simulink library "mysharedTrackingLibrary"  (R2023b)
settings: Solver=VariableStepAuto  StartTime=0.0  StopTime=10.0  RelTol=1e-3
undefined symbols (not defined in the file or in its folder): p
libraries: $bdroot x3
(part 2 of 2)

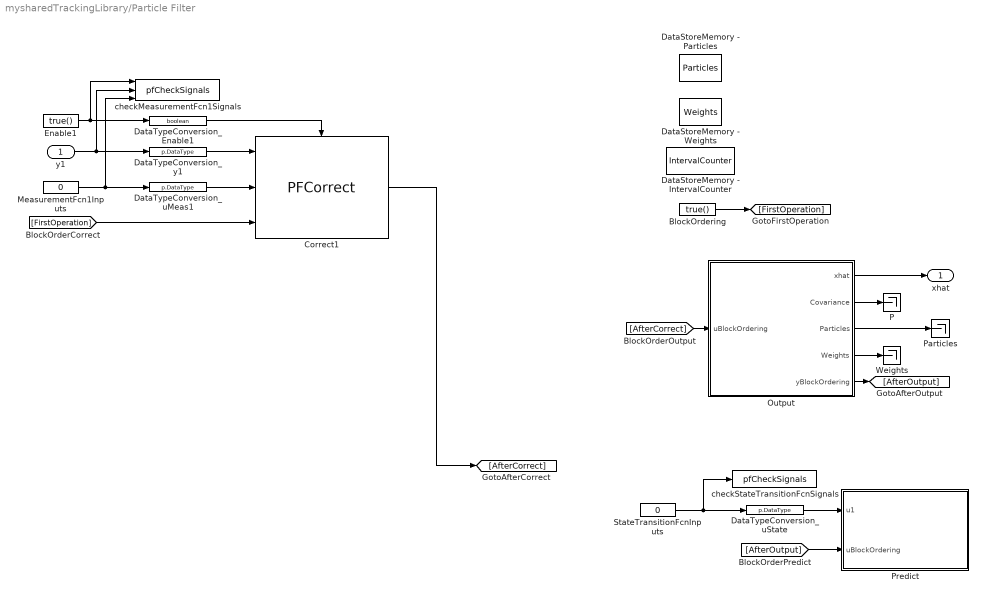
== system mysharedTrackingLibrary/Particle Filter ==
  y1 : Inport
  BlockOrdering : Constant  Value=true()  OutDataTypeStr=boolean
  Correct1 : $bdroot/Extras/PFCorrect  ProcessedMaskData=p
  DataStoreMemory - IntervalCounter : DataStoreMemory  DataStoreName=IntervalCounter  VectorParams1D=off  ShowAdditionalParam=off  OutDataTypeStr=p.DataType
  DataStoreMemory - Particles : DataStoreMemory  DataStoreName=Particles  InitialValue=p.Particles  VectorParams1D=off  ShowAdditionalParam=off  OutDataTypeStr=p.DataType
  DataStoreMemory - Weights : DataStoreMemory  DataStoreName=Weights  InitialValue=p.Weights  VectorParams1D=off  ShowAdditionalParam=off  OutDataTypeStr=p.DataType
  DataTypeConversion_Enable1 : DataTypeConversion  OutDataTypeStr=boolean  SaturateOnIntegerOverflow=off  RndMeth=Floor
  DataTypeConversion_uMeas1 : DataTypeConversion  OutDataTypeStr=p.DataType  SaturateOnIntegerOverflow=off  RndMeth=Floor
  DataTypeConversion_uState : DataTypeConversion  OutDataTypeStr=p.DataType  SaturateOnIntegerOverflow=off  RndMeth=Floor
  DataTypeConversion_y1 : DataTypeConversion  OutDataTypeStr=p.DataType  SaturateOnIntegerOverflow=off  RndMeth=Floor
  Enable1 : Constant  Value=true()  SampleTime=p.SampleTimes.MeasurementFcn(1)
  MeasurementFcn1Inputs : Constant  Value=0  OutDataTypeStr=p.DataType  SampleTime=p.SampleTimes.MeasurementFcn(1)
  Output : Subsystem  TreatAsAtomicUnit=on  SystemSampleTime=p.SampleTimes.Output  mask{ProcessedMaskData=p}
      mask init:
      | if strcmp(get_param(bdroot,'SimulationStatus'),'stopped')
      |     pOutputs = [];
      | else
      |     pOutputs = ...
      |         matlabshared.tracking.internal.blocks.maskInitializationFcnPFOutputs(ProcessedMaskData);
      | end
  P : Terminator
  Particles : Terminator
  Predict : Subsystem  TreatAsAtomicUnit=on  SystemSampleTime=p.SampleTimes.StateTransitionFcn  mask(PFPredict){ProcessedMaskData=p}
      mask init:
      | if strcmp(get_param(bdroot,'SimulationStatus'),'stopped')
      |     pS = [];
      |     SampleTime = [];
      |     DataType = [];
      |     SLFcnsToRegister = {};
      | else
      |     [pS,SampleTime] = ...
      |         matlabshared.tracking.internal.blocks.maskInitializationFcnPFPredictor(ProcessedMaskData);
      |     [DataType,SLFcnsToRegister] = ...
      |         matlabshared.tracking.internal.blocks.maskInitializationFcnRegisterSLFcn(ProcessedMaskData, pS);
      | end
  StateTransitionFcnInputs : Constant  Value=0  OutDataTypeStr=p.DataType  SampleTime=p.SampleTimes.StateTransitionFcn
  Weights : Terminator
  checkMeasurementFcn1Signals : S-Function  FunctionName=pfCheckSignals  Parameters=signalCheck.BlockPath, signalCheck.MeasurementFcn{1}.PortNames, signalCheck.MeasurementFcn{1}.SampleTime, signalCheck.DataType, signalCheck.MeasurementFcn{1}.PortDimensions  SFunctionDeploymentMode=off  EnableBusSupport=off
  checkStateTransitionFcnSignals : S-Function  FunctionName=pfCheckSignals  Parameters=signalCheck.BlockPath, signalCheck.StateTransitionFcn.PortNames, signalCheck.StateTransitionFcn.SampleTime, signalCheck.DataType, signalCheck.StateTransitionFcn.PortDimensions  SFunctionDeploymentMode=off  EnableBusSupport=off
  xhat : Outport  VectorParamsAs1DForOutWhenUnconnected=off
  wires:
  [AfterCorrect] -> Output/1(uBlockOrdering)
  Correct1/1 -> [AfterCorrect]
  [AfterOutput] -> Predict/2(uBlockOrdering)
  BlockOrdering/1 -> [FirstOperation]
  [FirstOperation] -> Correct1/3
  DataTypeConversion_y1/1 -> Correct1/1
  DataTypeConversion_uMeas1/1 -> Correct1/2
  Enable1/1 -> checkMeasurementFcn1Signals/1, DataTypeConversion_Enable1/1
  StateTransitionFcnInputs/1 -> checkStateTransitionFcnSignals/1, DataTypeConversion_uState/1
  MeasurementFcn1Inputs/1 -> checkMeasurementFcn1Signals/3, DataTypeConversion_uMeas1/1
  DataTypeConversion_uState/1 -> Predict/1(u1)
  DataTypeConversion_Enable1/1 -> Correct1/Enable
  Output/5(yBlockOrdering) -> [AfterOutput]
  Output/1(xhat) -> xhat/1
  Output/3(Particles) -> Particles/1
  Output/4(Weights) -> Weights/1
  Output/2(Covariance) -> P/1
  y1/1 -> DataTypeConversion_y1/1, checkMeasurementFcn1Signals/2

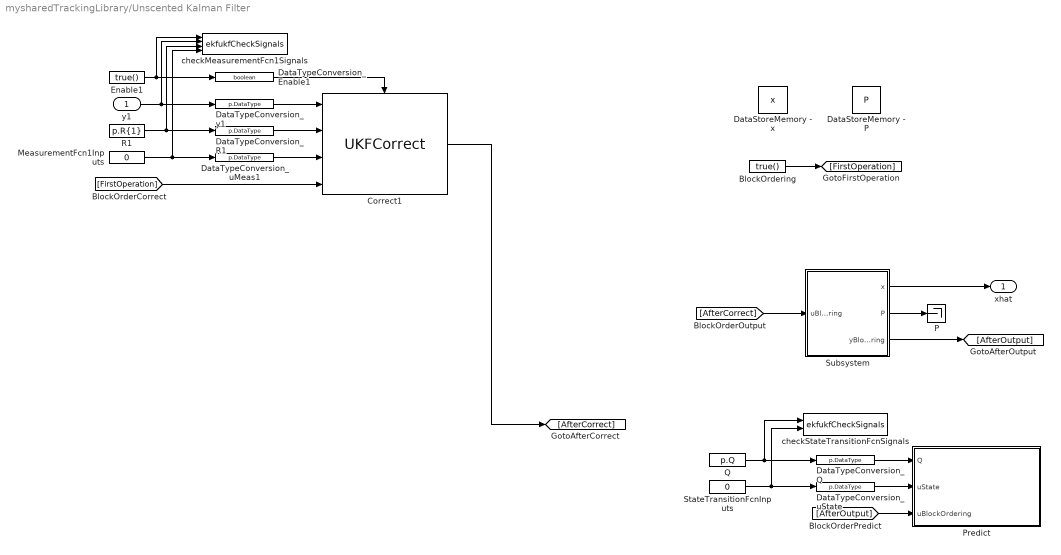
== system mysharedTrackingLibrary/Unscented Kalman Filter ==
  y1 : Inport
  BlockOrdering : Constant  Value=true()  OutDataTypeStr=boolean
  Correct1 : $bdroot/Extras/UKFCorrect  ProcessedMaskData=p
  DataStoreMemory - P : DataStoreMemory  DataStoreName=P  InitialValue=p.InitialCovariance  ShowAdditionalParam=off  OutDataTypeStr=p.DataType
  DataStoreMemory - x : DataStoreMemory  DataStoreName=x  InitialValue=p.InitialState  ShowAdditionalParam=off  OutDataTypeStr=p.DataType
  DataTypeConversion_Enable1 : DataTypeConversion  OutDataTypeStr=boolean  SaturateOnIntegerOverflow=off  RndMeth=Floor
  DataTypeConversion_Q : DataTypeConversion  OutDataTypeStr=p.DataType  SaturateOnIntegerOverflow=off  RndMeth=Floor
  DataTypeConversion_R1 : DataTypeConversion  OutDataTypeStr=p.DataType  SaturateOnIntegerOverflow=off  RndMeth=Floor
  DataTypeConversion_uMeas1 : DataTypeConversion  OutDataTypeStr=p.DataType  SaturateOnIntegerOverflow=off  RndMeth=Floor
  DataTypeConversion_uState : DataTypeConversion  OutDataTypeStr=p.DataType  SaturateOnIntegerOverflow=off  RndMeth=Floor
  DataTypeConversion_y1 : DataTypeConversion  OutDataTypeStr=p.DataType  SaturateOnIntegerOverflow=off  RndMeth=Floor
  Enable1 : Constant  Value=true()  SampleTime=p.SampleTimes.MeasurementFcn(1)
  MeasurementFcn1Inputs : Constant  Value=0  OutDataTypeStr=p.DataType  SampleTime=p.SampleTimes.MeasurementFcn(1)
  P : Terminator
  Predict : Subsystem  TreatAsAtomicUnit=on  SystemSampleTime=p.SampleTimes.StateTransitionFcn  mask(UKFPredict){ProcessedMaskData=p}
      mask init:
      | if strcmp(get_param(bdroot,'SimulationStatus'),'stopped')
      |     pS = [];
      |     SampleTime = [];
      |     DataType = [];
      |     SLFcnsToRegister = {};
      | else
      |     [pS,SampleTime] = ...
      |         matlabshared.tracking.internal.blocks.maskInitializationFcnUKFPredictor(ProcessedMaskData);
      |     [DataType,SLFcnsToRegister] = ...
      |         matlabshared.tracking.internal.blocks.maskInitializationFcnRegisterSLFcn(ProcessedMaskData, pS);
      | end
  Q : Constant  Value=p.Q  SampleTime=p.SampleTimes.StateTransitionFcn
  R1 : Constant  Value=p.R{1}  SampleTime=p.SampleTimes.MeasurementFcn(1)
  StateTransitionFcnInputs : Constant  Value=0  OutDataTypeStr=p.DataType  SampleTime=p.SampleTimes.StateTransitionFcn
  Subsystem : Subsystem  TreatAsAtomicUnit=on  SystemSampleTime=p.SampleTimes.Output
  checkMeasurementFcn1Signals : S-Function  FunctionName=ekfukfCheckSignals  Parameters=signalCheck.BlockPath, signalCheck.MeasurementFcn{1}.PortNames, signalCheck.MeasurementFcn{1}.SampleTime, signalCheck.DataType, signalCheck.MeasurementFcn{1}.PortDimensions, 1, signalCheck.MeasurementFcn{1}.HasAdditiveNoise  SFunctionDeploymentMode=off  EnableBusSupport=off
  checkStateTransitionFcnSignals : S-Function  FunctionName=ekfukfCheckSignals  Parameters=signalCheck.BlockPath, signalCheck.StateTransitionFcn.PortNames, signalCheck.StateTransitionFcn.SampleTime, signalCheck.DataType, signalCheck.StateTransitionFcn.PortDimensions, 0, signalCheck.StateTransitionFcn.HasAdditiveNoise  SFunctionDeploymentMode=off  EnableBusSupport=off
  xhat : Outport  VectorParamsAs1DForOutWhenUnconnected=off
  wires:
  [AfterOutput] -> Predict/3(uBlockOrdering)
  BlockOrdering/1 -> [FirstOperation]
  [FirstOperation] -> Correct1/4
  DataTypeConversion_y1/1 -> Correct1/1
  y1/1 -> checkMeasurementFcn1Signals/2, DataTypeConversion_y1/1
  R1/1 -> checkMeasurementFcn1Signals/3, DataTypeConversion_R1/1
  DataTypeConversion_uMeas1/1 -> Correct1/3
  Enable1/1 -> checkMeasurementFcn1Signals/1, DataTypeConversion_Enable1/1
  StateTransitionFcnInputs/1 -> checkStateTransitionFcnSignals/2, DataTypeConversion_uState/1
  MeasurementFcn1Inputs/1 -> checkMeasurementFcn1Signals/4, DataTypeConversion_uMeas1/1
  DataTypeConversion_R1/1 -> Correct1/2
  DataTypeConversion_uState/1 -> Predict/2(uState)
  Q/1 -> checkStateTransitionFcnSignals/1, DataTypeConversion_Q/1
  DataTypeConversion_Enable1/1 -> Correct1/Enable
  DataTypeConversion_Q/1 -> Predict/1(Q)
  [AfterCorrect] -> Subsystem/1(uBlockOrdering)
  Subsystem/1(x) -> xhat/1
  Subsystem/2(P) -> P/1
  Subsystem/3(yBlockOrdering) -> [AfterOutput]
  Correct1/1 -> [AfterCorrect]

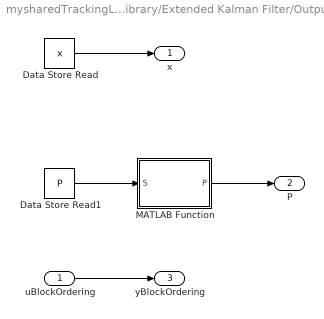
== system mysharedTrackingLibrary/Extended Kalman Filter/Output ==
  uBlockOrdering : Inport
  Data Store Read : DataStoreRead  DataStoreName=x  IndexOptions=Index vector (dialog)  Indices=1  OutputSizes=1
  Data Store Read1 : DataStoreRead  DataStoreName=P  IndexOptions=Index vector (dialog)  Indices=1  OutputSizes=1
  MATLAB Function : MATLAB Function  TreatAsAtomicUnit=on
  x : Outport  VectorParamsAs1DForOutWhenUnconnected=off
  P : Outport  Port=2  VectorParamsAs1DForOutWhenUnconnected=off
  yBlockOrdering : Outport  Port=3  VectorParamsAs1DForOutWhenUnconnected=off
  wires:
  Data Store Read/1 -> x/1
  Data Store Read1/1 -> MATLAB Function/1(S)
  uBlockOrdering/1 -> yBlockOrdering/1
  MATLAB Function/1(P) -> P/1

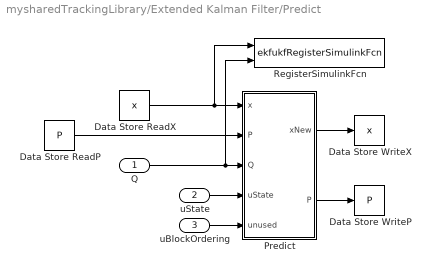
== system mysharedTrackingLibrary/Extended Kalman Filter/Predict ==
  Q : Inport  SampleTime=SampleTime
  uState : Inport  Port=2  SampleTime=SampleTime
  uBlockOrdering : Inport  Port=3  SampleTime=SampleTime
  Data Store WriteP : DataStoreWrite  DataStoreName=P  IndexOptions=Index vector (dialog)  Indices=1  OutputSizes=1
  Data Store WriteX : DataStoreWrite  DataStoreName=x  IndexOptions=Index vector (dialog)  Indices=1  OutputSizes=1
  Data Store ReadP : DataStoreRead  DataStoreName=P  IndexOptions=Index vector (dialog)  Indices=1  OutputSizes=1
  Data Store ReadX : DataStoreRead  DataStoreName=x  IndexOptions=Index vector (dialog)  Indices=1  OutputSizes=1
  Predict : MATLAB Function  TreatAsAtomicUnit=on
  RegisterSimulinkFcn : S-Function  FunctionName=ekfukfRegisterSimulinkFcn  Parameters=int32(2), 0, pS.HasAdditiveNoise, SampleTime, DataType, SLFcnsToRegister  SFunctionDeploymentMode=off  EnableBusSupport=off
  wires:
  Data Store ReadP/1 -> Predict/2("P ")
  Predict/2(P) -> Data Store WriteP/1
  Q/1 -> Predict/3(Q), RegisterSimulinkFcn/2
  Predict/1(xNew) -> Data Store WriteX/1
  Data Store ReadX/1 -> Predict/1(x), RegisterSimulinkFcn/1
  uBlockOrdering/1 -> Predict/5(unused)
  uState/1 -> Predict/4(uState)

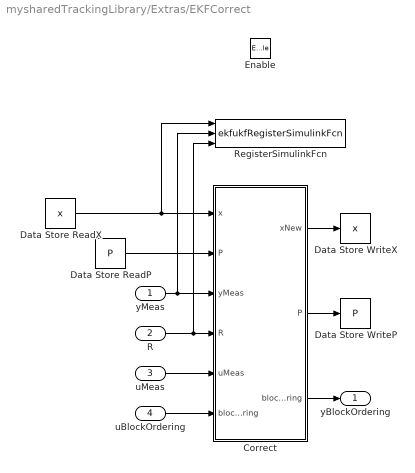
== system mysharedTrackingLibrary/Extras/EKFCorrect ==
  yMeas : Inport  SampleTime=SampleTime
  R : Inport  Port=2  SampleTime=SampleTime
  uMeas : Inport  Port=3  SampleTime=SampleTime
  uBlockOrdering : Inport  Port=4  SampleTime=SampleTime
  Enable : EnablePort
  Correct : MATLAB Function  TreatAsAtomicUnit=on
  Data Store ReadP : DataStoreRead  DataStoreName=P  IndexOptions=Index vector (dialog)  Indices=1  OutputSizes=1
  Data Store ReadX : DataStoreRead  DataStoreName=x  IndexOptions=Index vector (dialog)  Indices=1  OutputSizes=1
  Data Store WriteP : DataStoreWrite  DataStoreName=P  IndexOptions=Index vector (dialog)  Indices=1  OutputSizes=1
  Data Store WriteX : DataStoreWrite  DataStoreName=x  IndexOptions=Index vector (dialog)  Indices=1  OutputSizes=1
  RegisterSimulinkFcn : S-Function  FunctionName=ekfukfRegisterSimulinkFcn  Parameters=int32(3), 1, pM.HasAdditiveNoise, SampleTime, DataType, SLFcnsToRegister  SFunctionDeploymentMode=off  EnableBusSupport=off
  yBlockOrdering : Outport  VectorParamsAs1DForOutWhenUnconnected=off
  wires:
  Data Store ReadX/1 -> RegisterSimulinkFcn/1, Correct/1(x)
  Data Store ReadP/1 -> Correct/2("P ")
  Correct/2(P) -> Data Store WriteP/1
  yMeas/1 -> Correct/3(yMeas), RegisterSimulinkFcn/2
  R/1 -> Correct/4(R), RegisterSimulinkFcn/3
  Correct/1(xNew) -> Data Store WriteX/1
  Correct/3(blockOrdering) -> yBlockOrdering/1
  uBlockOrdering/1 -> Correct/6("blockOrdering ")
  uMeas/1 -> Correct/5(uMeas)

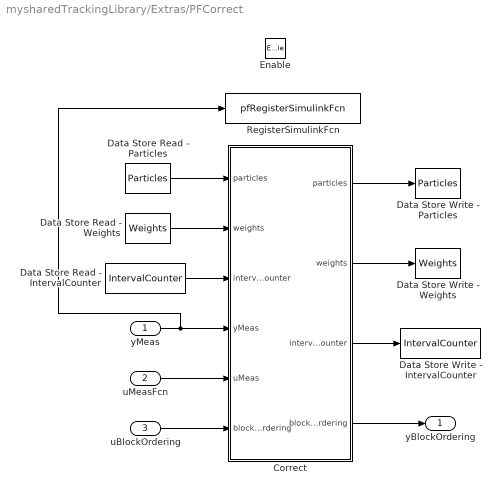
== system mysharedTrackingLibrary/Extras/PFCorrect ==
  yMeas : Inport  SampleTime=SampleTime
  uMeasFcn : Inport  Port=2  SampleTime=SampleTime
  uBlockOrdering : Inport  Port=3  SampleTime=SampleTime
  Enable : EnablePort
  Correct : MATLAB Function  TreatAsAtomicUnit=on
  Data Store Read - IntervalCounter : DataStoreRead  DataStoreName=IntervalCounter  IndexOptions=Index vector (dialog)  Indices=1  OutputSizes=1
  Data Store Read - Particles : DataStoreRead  DataStoreName=Particles  IndexOptions=Index vector (dialog)  Indices=1  OutputSizes=1
  Data Store Read - Weights : DataStoreRead  DataStoreName=Weights  IndexOptions=Index vector (dialog)  Indices=1  OutputSizes=1
  Data Store Write - IntervalCounter : DataStoreWrite  DataStoreName=IntervalCounter  IndexOptions=Index vector (dialog)  Indices=1  OutputSizes=1
  Data Store Write - Particles : DataStoreWrite  DataStoreName=Particles  IndexOptions=Index vector (dialog)  Indices=1  OutputSizes=1
  Data Store Write - Weights : DataStoreWrite  DataStoreName=Weights  IndexOptions=Index vector (dialog)  Indices=1  OutputSizes=1
  RegisterSimulinkFcn : S-Function  FunctionName=pfRegisterSimulinkFcn  Parameters=int32(1), 1, SampleTime, pRegisterSLFcn.DataType, pRegisterSLFcn.SLFcnsToRegister, pRegisterSLFcn.NumStates, pRegisterSLFcn.NumParticles, pRegisterSLFcn.IsStateOrientationColumn  SFunctionDeploymentMode=off  EnableBusSupport=off
  yBlockOrdering : Outport  VectorParamsAs1DForOutWhenUnconnected=off
  wires:
  Data Store Read - Particles/1 -> Correct/1("particles ")
  yMeas/1 -> RegisterSimulinkFcn/1, Correct/4(yMeas)
  Correct/1(particles) -> Data Store Write - Particles/1
  uBlockOrdering/1 -> Correct/6("blockOrdering ")
  Correct/4(blockOrdering) -> yBlockOrdering/1
  Data Store Read - Weights/1 -> Correct/2("weights ")
  Correct/2(weights) -> Data Store Write - Weights/1
  Correct/3(intervalCounter) -> Data Store Write - IntervalCounter/1
  Data Store Read - IntervalCounter/1 -> Correct/3("intervalCounter ")
  uMeasFcn/1 -> Correct/5(uMeas)

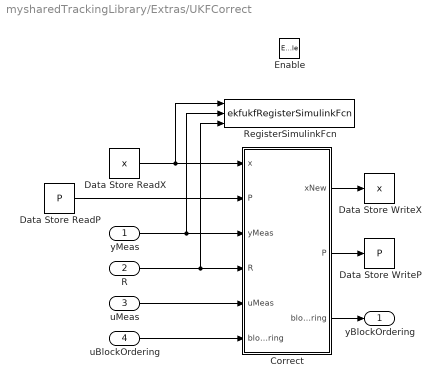
== system mysharedTrackingLibrary/Extras/UKFCorrect ==
  yMeas : Inport  SampleTime=SampleTime
  R : Inport  Port=2  SampleTime=SampleTime
  uMeas : Inport  Port=3  SampleTime=SampleTime
  uBlockOrdering : Inport  Port=4  SampleTime=SampleTime
  Enable : EnablePort
  Correct : MATLAB Function  TreatAsAtomicUnit=on
  Data Store WriteP : DataStoreWrite  DataStoreName=P  IndexOptions=Index vector (dialog)  Indices=1  OutputSizes=1
  Data Store WriteX : DataStoreWrite  DataStoreName=x  IndexOptions=Index vector (dialog)  Indices=1  OutputSizes=1
  Data Store ReadP : DataStoreRead  DataStoreName=P  IndexOptions=Index vector (dialog)  Indices=1  OutputSizes=1
  Data Store ReadX : DataStoreRead  DataStoreName=x  IndexOptions=Index vector (dialog)  Indices=1  OutputSizes=1
  RegisterSimulinkFcn : S-Function  FunctionName=ekfukfRegisterSimulinkFcn  Parameters=int32(3), 1, pM.HasAdditiveNoise, SampleTime, DataType, SLFcnsToRegister  SFunctionDeploymentMode=off  EnableBusSupport=off
  yBlockOrdering : Outport  VectorParamsAs1DForOutWhenUnconnected=off
  wires:
  Data Store ReadX/1 -> Correct/1(x), RegisterSimulinkFcn/1
  Data Store ReadP/1 -> Correct/2("P ")
  Correct/2(P) -> Data Store WriteP/1
  yMeas/1 -> RegisterSimulinkFcn/2, Correct/3(yMeas)
  R/1 -> Correct/4(R), RegisterSimulinkFcn/3
  Correct/1(xNew) -> Data Store WriteX/1
  uBlockOrdering/1 -> Correct/6("blockOrdering ")
  Correct/3(blockOrdering) -> yBlockOrdering/1
  uMeas/1 -> Correct/5(uMeas)

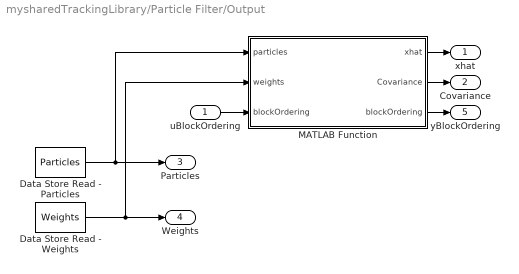
== system mysharedTrackingLibrary/Particle Filter/Output ==
  uBlockOrdering : Inport
  Data Store Read - Particles : DataStoreRead  DataStoreName=Particles  IndexOptions=Index vector (dialog)  Indices=1  OutputSizes=1
  Data Store Read - Weights : DataStoreRead  DataStoreName=Weights  IndexOptions=Index vector (dialog)  Indices=1  OutputSizes=1
  MATLAB Function : MATLAB Function  TreatAsAtomicUnit=on
  xhat : Outport  VectorParamsAs1DForOutWhenUnconnected=off
  Covariance : Outport  Port=2  VectorParamsAs1DForOutWhenUnconnected=off
  Particles : Outport  Port=3  VectorParamsAs1DForOutWhenUnconnected=off
  Weights : Outport  Port=4  VectorParamsAs1DForOutWhenUnconnected=off
  yBlockOrdering : Outport  Port=5  VectorParamsAs1DForOutWhenUnconnected=off
  wires:
  Data Store Read - Weights/1 -> Weights/1, MATLAB Function/2(weights)
  Data Store Read - Particles/1 -> MATLAB Function/1(particles), Particles/1
  MATLAB Function/2(Covariance) -> Covariance/1
  MATLAB Function/1(xhat) -> xhat/1
  uBlockOrdering/1 -> MATLAB Function/3("blockOrdering ")
  MATLAB Function/3(blockOrdering) -> yBlockOrdering/1

== system mysharedTrackingLibrary/Particle Filter/Predict ==
  u1 : Inport  SampleTime=SampleTime
  uBlockOrdering : Inport  Port=2  SampleTime=SampleTime
  Data Store Read - Particles : DataStoreRead  DataStoreName=Particles  IndexOptions=Index vector (dialog)  Indices=1  OutputSizes=1
  Data Store Write - Particles : DataStoreWrite  DataStoreName=Particles  IndexOptions=Index vector (dialog)  Indices=1  OutputSizes=1
  Predict : MATLAB Function  TreatAsAtomicUnit=on
  RegisterSimulinkFcn : S-Function  FunctionName=pfRegisterSimulinkFcn  Parameters=int32(1), 0, SampleTime, DataType, SLFcnsToRegister, pS.NumStates, pS.NumParticles, pS.IsStateOrientationColumn  SFunctionDeploymentMode=off  EnableBusSupport=off
  wires:
  Predict/1(predictedParticles) -> Data Store Write - Particles/1
  Data Store Read - Particles/1 -> RegisterSimulinkFcn/1, Predict/1(particles)
  uBlockOrdering/1 -> Predict/3(unused)
  u1/1 -> Predict/2(uState)

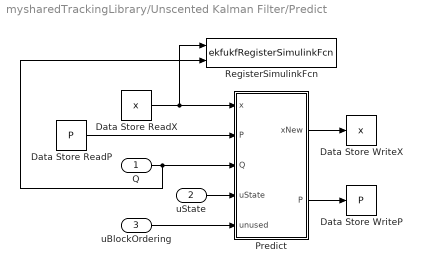
== system mysharedTrackingLibrary/Unscented Kalman Filter/Predict ==
  Q : Inport  SampleTime=SampleTime
  uState : Inport  Port=2  SampleTime=SampleTime
  uBlockOrdering : Inport  Port=3  SampleTime=SampleTime
  Data Store WriteP : DataStoreWrite  DataStoreName=P  IndexOptions=Index vector (dialog)  Indices=1  OutputSizes=1
  Data Store WriteX : DataStoreWrite  DataStoreName=x  IndexOptions=Index vector (dialog)  Indices=1  OutputSizes=1
  Data Store ReadP : DataStoreRead  DataStoreName=P  IndexOptions=Index vector (dialog)  Indices=1  OutputSizes=1
  Data Store ReadX : DataStoreRead  DataStoreName=x  IndexOptions=Index vector (dialog)  Indices=1  OutputSizes=1
  Predict : MATLAB Function  TreatAsAtomicUnit=on
  RegisterSimulinkFcn : S-Function  FunctionName=ekfukfRegisterSimulinkFcn  Parameters=int32(2), 0, pS.HasAdditiveNoise, SampleTime, DataType, SLFcnsToRegister  SFunctionDeploymentMode=off  EnableBusSupport=off
  wires:
  Data Store ReadP/1 -> Predict/2("P ")
  Predict/2(P) -> Data Store WriteP/1
  Q/1 -> RegisterSimulinkFcn/2, Predict/3(Q)
  Predict/1(xNew) -> Data Store WriteX/1
  Data Store ReadX/1 -> Predict/1(x), RegisterSimulinkFcn/1
  uBlockOrdering/1 -> Predict/5(unused)
  uState/1 -> Predict/4(uState)

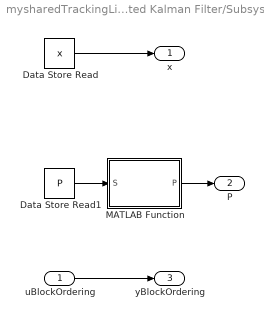
== system mysharedTrackingLibrary/Unscented Kalman Filter/Subsystem ==
  uBlockOrdering : Inport
  Data Store Read : DataStoreRead  DataStoreName=x  IndexOptions=Index vector (dialog)  Indices=1  OutputSizes=1
  Data Store Read1 : DataStoreRead  DataStoreName=P  IndexOptions=Index vector (dialog)  Indices=1  OutputSizes=1
  MATLAB Function : MATLAB Function  TreatAsAtomicUnit=on
  x : Outport  VectorParamsAs1DForOutWhenUnconnected=off
  P : Outport  Port=2  VectorParamsAs1DForOutWhenUnconnected=off
  yBlockOrdering : Outport  Port=3  VectorParamsAs1DForOutWhenUnconnected=off
  wires:
  Data Store Read/1 -> x/1
  Data Store Read1/1 -> MATLAB Function/1(S)
  uBlockOrdering/1 -> yBlockOrdering/1
  MATLAB Function/1(P) -> P/1

== matlab function mysharedTrackingLibrary/Particle Filter/Predict/Predict ==
  settings: updateMethod=DISCRETE  sampleTime=SampleTime
  data: particles input; predictedParticles output; uState input; unused input; pS parameter
function predictedParticles = pfPredict(particles,uState,~,pS)
% pfPredict Prediction step for particle filter
%
% Inputs:
%    particles - Particles before prediction
%    pS        - Structure containing nontunable parameters
%                 FcnName - Name of the state transition fcn, a Simulink fcn
%                 IsStateOrientationColumn - particles is [Ns Np] if true
%                                            particles is [Np Ns] if false
%                 IsStateVariableCircular - [1 Ns] logical array. Indicates
%                                           the circular states
%
%   Copyright 2017 The MathWorks, Inc.

%#codegen

if pS.IsSimulinkFcn
    fcnH_SL = str2func(pS.FcnName);
    fcnH = @(fParticles)fcnH_SL(fParticles);
else
    fcnH = str2func(pS.FcnName);
end
switch pS.NumberOfExtraArgumentInports
    case 0
        extraArgs = {};
    case 1
        extraArgs = {uState};
    otherwise
        assert(false);
end

predictedParticles = matlabshared.tracking.internal.ParticleFilter.pfBlockPredict(fcnH,particles,pS,extraArgs{:});
end

== matlab function mysharedTrackingLibrary/Particle Filter/Output/MATLAB Function ==
  data: particles input; weights input; blockOrdering input; pOutputs parameter; xhat output; Covariance output; blockOrdering output
function [xhat,Covariance,blockOrdering] = ...
    calculateStateAndCovariance(particles,weights,blockOrdering,pOutputs)

%% Quick return if no work is needed
if strcmp(pOutputs.StateEstimationMethod,'none')
    xhat = cast(0,'like',particles);
    Covariance = cast(0,'like',particles);
    return;
end

%% Preparation
% Get the state estimator object
switch pOutputs.StateEstimationMethod
    case 'mean'
        stateEstimator = matlabshared.tracking.internal.MeanStateEstimator;
        OutputState = true();
        OutputCov = pOutputs.OutputStateCovariance; % Follow user's preference
    case 'maxweight'
        stateEstimator = matlabshared.tracking.internal.MaxWeightStateEstimator;
        OutputState = true();
        OutputCov = false(); % No covariance to output, even if user requested
    case 'none'
        % This code path should never be reached due to quick return code
        % in the beginnin
        stateEstimator = cast(0,'like',particles);
        OutputState = false();
        OutputCov = false();
    otherwise
        assert(false);
end
% Get the particle manager
particleManager = matlabshared.tracking.internal.ParticleFilter.initializeParticleManager(pOutputs.IsStateOrientationColumn);

%% Results
% At least 1 output was requested (Covariance or xhat)   
if OutputCov
    % xhat is calculated in the process of calculating Covariance. No need
    % to check if xhat was requested or not. Block will not show an outport
    % if xhat was not requested.
    [xhat,Covariance] = stateEstimator.estimate(particleManager, particles,...
        weights, pOutputs.IsStateVariableCircular);
elseif OutputState
    % xhat was requested, but not the covariance. 
    xhat = stateEstimator.estimate(particleManager, particles, weights,...
        pOutputs.IsStateVariableCircular);
    Covariance = cast(0,'like',particles);
else
    xhat = cast(0,'like',particles);
    Covariance = cast(0,'like',particles);
end

end

== matlab function mysharedTrackingLibrary/Extras/UKFCorrect/Correct ==
  settings: updateMethod=DISCRETE  sampleTime=SampleTime
  data: x input; xNew output; P input; P output; yMeas input; R input; uMeas input; blockOrdering input; pM parameter; blockOrdering output
function [xNew,P,blockOrdering] = ukfCorrect(x,P,yMeas,R,uMeas,blockOrdering,pM)
% ukfCorrect Correction step for UKF
%
%   Copyright 2016-2021 The MathWorks, Inc.

%#codegen

% If measurement noise is time-varying then compute square-root
% factorization.
if pM.HasTimeVaryingR
   R = matlabshared.tracking.internal.svdPSD(R);
end

% Construct the function handle for measurement fcn
if pM.IsSimulinkFcn
    MeasurementFcnH_SL = str2func(pM.FcnName);
    if pM.HasAdditiveNoise
        MeasurementFcnH = @(fState)MeasurementFcnH_SL(fState);
    else
        MeasurementFcnH = @(fState,fMeasNoise)MeasurementFcnH_SL(fState,fMeasNoise);
    end
else
    MeasurementFcnH = str2func(pM.FcnName);
end

% Handle (optional) extra input arguments of the measurement fcn
switch pM.NumberOfExtraArgumentInports
    case 0
        extraArgs = {};
    case 1
        extraArgs = {uMeas};
    otherwise
        assert(false);
end

% Construct the corrector, perform the update
if pM.HasAdditiveNoise
    ukfCorrector = matlabshared.tracking.internal.UKFCorrectorAdditive();
    
    % MeasurementFcn
    ztry = MeasurementFcnH(x, extraArgs{:});   
else
    ukfCorrector = matlabshared.tracking.internal.UKFCorrectorNonAdditive();
    
    % MeasurementFcn
    ztry = MeasurementFcnH(...
       x, zeros(size(R,1),1,'like',x), ...
       extraArgs{:});
end

if pM.IsSimulinkFcn
   hasError = (numel(ztry) ~= numel(yMeas));
else
   hasError = (numel(ztry) ~= numel(yMeas)) || ~isa(ztry, class(x));
end

coder.internal.errorIf(...
   hasError,...
   'shared_tracking:UnscentedKalmanFilter:MeasurementNonMatchingSizeOrClass',...
   'MeasurementFcn');

% Measurement wrapping
ukfCorrector.HasMeasurementWrapping = pM.HasWrapping;

xNew = zeros(size(x),'like',x); %#ok<PREALL>
[xNew, P] = ukfCorrector.correct(...
        yMeas,R,x,P,...
        pM.Alpha, pM.Beta, pM.Kappa,...
        MeasurementFcnH,extraArgs{:});
end

== matlab function mysharedTrackingLibrary/Unscented Kalman Filter/Predict/Predict ==
  settings: updateMethod=DISCRETE  sampleTime=SampleTime
  data: x input; xNew output; P input; Q input; uState input; unused input; P output; pS parameter
function [xNew,P] = ukfPredict(x,P,Q,uState,~,pS)
% ukfCorrect Prediction step for UKF
%
%   Copyright 2016-2021 The MathWorks, Inc.

%#codegen

% If process noise is time-varying then compute square-root
% factorization.
if pS.HasTimeVaryingQ
   Q = matlabshared.tracking.internal.svdPSD(Q);
end

if pS.IsSimulinkFcn
    StateTransitionFcnH_SL = str2func(pS.FcnName);
    if pS.HasAdditiveNoise
        StateTransitionFcnH = @(fState)StateTransitionFcnH_SL(fState);
    else
        StateTransitionFcnH = @(fState,fProcNoise)StateTransitionFcnH_SL(fState,fProcNoise);
    end
else
    StateTransitionFcnH = str2func(pS.FcnName);
end
switch pS.NumberOfExtraArgumentInports
    case 0
        extraArgs = {};
    case 1
        extraArgs = {uState};
    otherwise
        assert(false);
end

xNew = zeros(size(x),'like',x); %#ok<PREALL>
if pS.HasAdditiveNoise
   % Additive noise
   
   % StateTransitionFcn
   xTry = StateTransitionFcnH(x, extraArgs{:});
  
   if pS.IsSimulinkFcn
      hasError = any(size(x) ~= size(xTry));
   else
      hasError = any(size(x) ~= size(xTry)) || ~isa(xTry, class(x));
   end
   
   coder.internal.errorIf(...
      hasError,...
      'shared_tracking:UnscentedKalmanFilter:StateNonMatchingSizeOrClass',...
      'StateTransitionFcn', 'State', numel(x));
   
    [xNew,P] = matlabshared.tracking.internal.UKFPredictorAdditive.predict(...
        Q,x,P,...
        pS.Alpha, pS.Beta, pS.Kappa,...
        StateTransitionFcnH, extraArgs{:});
else 
   % Non-additive noise
   
   % StateTransitionFcn
   xTry = StateTransitionFcnH(x, zeros(size(Q,1),1,'like',x),extraArgs{:});
   
   if pS.IsSimulinkFcn
      hasError = any(size(x) ~= size(xTry));
   else
      hasError = any(size(x) ~= size(xTry)) || ~isa(xTry, class(x));
   end
   
   coder.internal.errorIf(...
      hasError,...
      'shared_tracking:UnscentedKalmanFilter:StateNonMatchingSizeOrClass',...
      'StateTransitionFcn', 'State', numel(x));
   
    [xNew,P] = matlabshared.tracking.internal.UKFPredictorNonAdditive.predict(...
        Q,x,P,...
        pS.Alpha, pS.Beta, pS.Kappa,...
        StateTransitionFcnH, extraArgs{:});    
end
end

== matlab function mysharedTrackingLibrary/Extended Kalman Filter/Output/MATLAB Function ==
  data: S input; P output
function P = fcn(S)
    
    % Get back Covariance from Square-root Covariance
    P = S*S';
    
end

== matlab function mysharedTrackingLibrary/Unscented Kalman Filter/Subsystem/MATLAB Function ==
  data: S input; P output
function P = fcn(S)
    
    % Get back Covariance from Square-root Covariance
    P = S*S';
    
end

== matlab function mysharedTrackingLibrary/Extras/EKFCorrect/Correct ==
  settings: updateMethod=DISCRETE  sampleTime=SampleTime
  data: x input; xNew output; P input; P output; yMeas input; R input; uMeas input; blockOrdering input; pM parameter; blockOrdering output
function [xNew,P,blockOrdering] = fcn(x,P,yMeas,R,uMeas,blockOrdering,pM)
% ekfCorrect Correction step for EKF
%
%   Copyright 2016-2021 The MathWorks, Inc.

%#codegen

% If measurement noise is time-varying then compute square-root
% factorization.
if pM.HasTimeVaryingR
   R = matlabshared.tracking.internal.svdPSD(R);
end

% Construct the function handle for measurement fcn
if pM.IsSimulinkFcn
    MeasurementFcnH_SL = str2func(pM.FcnName);
    if pM.HasAdditiveNoise
        MeasurementFcnH = @(fState)MeasurementFcnH_SL(fState);
    else
        MeasurementFcnH = @(fState,fMeasNoise)MeasurementFcnH_SL(fState,fMeasNoise);
    end
else
    MeasurementFcnH = str2func(pM.FcnName);
end

% Construct the function handle for measurement Jacobian fcn
if pM.HasJacobian
    if pM.IsSimulinkFcn
        MeasurementJacobianFcnH_SL = str2func(pM.JacobianFcnName);
        if pM.HasAdditiveNoise
            MeasurementJacobianFcnH = @(fState)MeasurementJacobianFcnH_SL(fState);
        else
            MeasurementJacobianFcnH = @(fState,fMeasNoise)MeasurementJacobianFcnH_SL(fState,fMeasNoise);
        end
    else
        MeasurementJacobianFcnH = str2func(pM.JacobianFcnName);
    end
else
    MeasurementJacobianFcnH = [];
end

% Handle (optional) extra input arguments of the measurement & jacobian fcns
switch pM.NumberOfExtraArgumentInports
    case 0
        extraArgs = {};
    case 1
        extraArgs = {uMeas};
    otherwise
        assert(false);
end

% Construct the corrector, perform the update
if pM.HasAdditiveNoise
    ekfCorrector = matlabshared.tracking.internal.EKFCorrectorAdditive();
else
    ekfCorrector = matlabshared.tracking.internal.EKFCorrectorNonAdditive();
end

% Check if dimensions and type of Measurement and Jacobian are correct
if pM.HasAdditiveNoise
   % Additive noise
   
   % MeasurementFcn
   ztry = MeasurementFcnH(x, extraArgs{:});
   
   if pM.IsSimulinkFcn
      hasError = (numel(ztry) ~= numel(yMeas));
   else
      hasError = (numel(ztry) ~= numel(yMeas)) || ~isa(ztry, class(x));
   end
   
   coder.internal.errorIf(...
      hasError,...
      'shared_tracking:ExtendedKalmanFilter:MeasurementNonMatchingSizeOrClass',...
      'MeasurementFcn');
   
   if pM.HasJacobian
      % MeasurementJacobianFcn
      Htry = MeasurementJacobianFcnH(x, extraArgs{:});
      isSizeNotCorrect = numel(yMeas) ~= size(Htry,1) || numel(x) ~= size(Htry,2);
      
      if pM.IsSimulinkFcn
         hasError = isSizeNotCorrect;
      else
         hasError = isSizeNotCorrect || ~isa(Htry, class(x));
      end
      
      coder.internal.errorIf(...
         hasError,...
         'shared_tracking:ExtendedKalmanFilter:MeasurementJacobianNonMatchingSizeOrClass',...
         'MeasurementJacobianFcn',numel(yMeas),numel(x));
   end   
else
   % Non-additive noise
   
   % MeasurementFcn
   ztry = MeasurementFcnH(...
      x, zeros(size(R,1),1,'like',x), ...
      extraArgs{:});   

   if pM.IsSimulinkFcn
      hasError = (numel(ztry) ~= numel(yMeas));
   else
      hasError = (numel(ztry) ~= numel(yMeas)) || ~isa(ztry, class(x));
   end
   
   coder.internal.errorIf(...
      hasError,...
      'shared_tracking:ExtendedKalmanFilter:MeasurementNonMatchingSizeOrClass',...
      'MeasurementFcn');
   
   if pM.HasJacobian
      % MeasurementJacobianFcn
      Htry = MeasurementJacobianFcnH(...
         x, zeros(size(R,1),1,'like',x), ...
         extraArgs{:});
      
      isSizeNotCorrect = numel(yMeas) ~= size(Htry,1) || numel(x) ~= size(Htry,2);     
      
      if pM.IsSimulinkFcn
         hasError = isSizeNotCorrect;
      else
         hasError = isSizeNotCorrect || ~isa(Htry, class(x));
      end
      
      coder.internal.errorIf(...
         hasError,...
         'shared_tracking:ExtendedKalmanFilter:MeasurementJacobianNonMatchingSizeOrClass',...
         'MeasurementJacobianFcn',numel(yMeas),numel(x));
   end
end
% Measurement wrapping
ekfCorrector.HasMeasurementWrapping = pM.HasWrapping;

xNew = zeros(size(x),'like',x); %#ok<PREALL>

[xNew,P] = ekfCorrector.correct(...
        yMeas,R,x,P,MeasurementFcnH,MeasurementJacobianFcnH,extraArgs{:});
end

== matlab function mysharedTrackingLibrary/Extended Kalman Filter/Predict/Predict ==
  settings: updateMethod=DISCRETE  sampleTime=SampleTime
  data: x input; xNew output; P input; Q input; uState input; unused input; P output; pS parameter
function [xNew,P] = fcn(x,P,Q,uState,~,pS)
% ekfCorrect Prediction step for EKF
%
%   Copyright 2016-2021 The MathWorks, Inc.

%#codegen

% If process noise is time-varying then compute square-root
% factorization.
if pS.HasTimeVaryingQ
   Q = matlabshared.tracking.internal.svdPSD(Q);
end

% Construct fcn handles
if pS.IsSimulinkFcn
    StateTransitionJacobianFcnH_SL = str2func(pS.FcnName);
    if pS.HasAdditiveNoise
        StateTransitionFcnH = @(fState)StateTransitionJacobianFcnH_SL(fState);
    else
        StateTransitionFcnH = @(fState,fProcNoise)StateTransitionJacobianFcnH_SL(fState,fProcNoise);
    end
else
    StateTransitionFcnH = str2func(pS.FcnName);
end
if pS.HasJacobian
    if pS.IsSimulinkFcn
        StateTransitionJacobianFcnH_SL = str2func(pS.JacobianFcnName);
        if pS.HasAdditiveNoise
            StateTransitionJacobianFcnH = @(fState)StateTransitionJacobianFcnH_SL(fState);
        else
            StateTransitionJacobianFcnH = @(fState,fProcNoise)StateTransitionJacobianFcnH_SL(fState,fProcNoise);
        end
    else
        StateTransitionJacobianFcnH = str2func(pS.JacobianFcnName);
    end
else
    StateTransitionJacobianFcnH = [];
end

switch pS.NumberOfExtraArgumentInports
    case 0
        extraArgs = {};
    case 1
        extraArgs = {uState};
    otherwise
        assert(false);
end

% Check if dimensions and type of State and Jacobian are correct
if pS.HasAdditiveNoise
   % Additive noise
   
   % StateTransitionFcn
   xTry = StateTransitionFcnH(x, extraArgs{:});
   
   if pS.IsSimulinkFcn
      hasError = any(size(x) ~= size(xTry));
   else
      hasError = any(size(x) ~= size(xTry)) || ~isa(xTry, class(x));
   end
   
   coder.internal.errorIf(...
      hasError,...
      'shared_tracking:ExtendedKalmanFilter:StateNonMatchingSizeOrClass',...
      'StateTransitionFcn', 'State', numel(x));
   
   if pS.HasJacobian
      % Jacobian
      F = StateTransitionJacobianFcnH(x, extraArgs{:});
      % F needs to be square
      isSizeNotCorrect = ~all(size(F) == numel(x));
      
      if pS.IsSimulinkFcn
         hasError = isSizeNotCorrect;
      else
         hasError = isSizeNotCorrect || ~isa(F, class(x));
      end
      
      coder.internal.errorIf(...
         hasError,...
         'shared_tracking:ExtendedKalmanFilter:StateTransitionJacobianNonMatchingSizeOrClass',...
         'StateTransitionJacobianFcn', numel(x));
   end
else
   % Non-additive noise
   
   % StateTransitionFcn
   xTry = StateTransitionFcnH(x, zeros(size(Q,1),1,'like',x),extraArgs{:});
   
   if pS.IsSimulinkFcn
      hasError = any(size(x) ~= size(xTry));
   else
      hasError = any(size(x) ~= size(xTry)) || ~isa(xTry, class(x));
   end
   
   coder.internal.errorIf(...
      hasError,...
      'shared_tracking:ExtendedKalmanFilter:StateNonMatchingSizeOrClass',...
      'StateTransitionFcn', 'State', numel(x))
   
   if pS.HasJacobian
      % Jacobian
      F = StateTransitionJacobianFcnH(x, zeros(size(Q,1),1,'like',x),extraArgs{:});
      % F needs to be square
      isSizeNotCorrect = ~all(size(F) == numel(x));
      
      if pS.IsSimulinkFcn
         hasError = isSizeNotCorrect;
      else
         hasError = isSizeNotCorrect || ~isa(F, class(x));
      end
       
      coder.internal.errorIf(...
         hasError,...
         'shared_tracking:ExtendedKalmanFilter:StateTransitionJacobianNonMatchingSizeOrClass',...
         'StateTransitionJacobianFcn', numel(x));
   end
end

xNew = zeros(size(x),'like',x); %#ok<PREALL>

if pS.HasAdditiveNoise
    [xNew,P] = matlabshared.tracking.internal.EKFPredictorAdditive.predict(...
        Q,x,P,StateTransitionFcnH,StateTransitionJacobianFcnH,extraArgs{:});
else    
    [xNew,P] = matlabshared.tracking.internal.EKFPredictorNonAdditive.predict(...
        Q,x,P,StateTransitionFcnH,StateTransitionJacobianFcnH,extraArgs{:});
end
end

== matlab function mysharedTrackingLibrary/Extras/PFCorrect/Correct ==
  settings: updateMethod=DISCRETE  sampleTime=SampleTime
  data: particles input; weights input; intervalCounter input; particles output; weights output; intervalCounter output; yMeas input; uMeas input; blockOrdering input; pM parameter; blockOrdering output
function [particles,weights,intervalCounter,blockOrdering] = ...
    pfCorrect(particles,weights,intervalCounter,yMeas,uMeas,blockOrdering,pM)
% pfCorrect Correction and resampling step for particle filter
%
%   Copyright 2017 The MathWorks, Inc.

%#codegen

persistent rngState;
if isempty(rngState)
    rng(pM.Seed,pM.RandomNumberGenerator);
    rngState = rng();
else
    rng(rngState);
end

if pM.IsSimulinkFcn
    fcnH_SL = str2func(pM.FcnName);
    fcnH = @(fParticles,fMeasurement)fcnH_SL(fParticles,fMeasurement);
else
    fcnH = str2func(pM.FcnName);
end
switch pM.NumberOfExtraArgumentInports
    case 0
        extraArgs = {};
    case 1
        extraArgs = {uMeas};
    otherwise
        assert(false);
end

[particles,weights,intervalCounter] = ...
    matlabshared.tracking.internal.ParticleFilter.pfBlockCorrectAndResample(...
    fcnH, particles, weights,intervalCounter,yMeas,pM,extraArgs{:});

rngState = rng();
end
